simulink model "ARX_model_and_real_data"  (Simulink 5.0)
settings: Solver=ode45  StartTime=0.0  StopTime=10.0  RelTol=1e-3
settings Model: LastModifiedBy=Admin

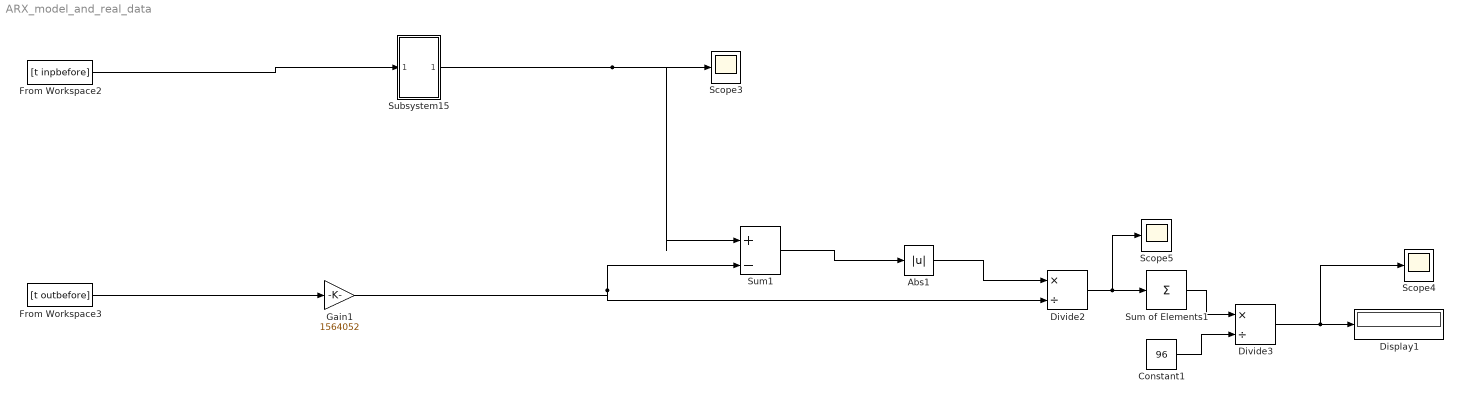
== system ARX_model_and_real_data ==
  Abs1 : Abs  SaturateOnIntegerOverflow=on
  Constant1 : Constant  Value=96
  Display1 : Display
  Divide2 : Product  Inputs=*/  ShowAdditionalParam=on  OutDataTypeMode=double  OutScaling=2^-10
  Divide3 : Product  Inputs=*/  ShowAdditionalParam=on  OutDataTypeMode=double  OutScaling=2^-10
  From Workspace2 : FromWorkspace  VariableName=[t inpbefore]  SampleTime=0
  From Workspace3 : FromWorkspace  VariableName=[t outbefore]  SampleTime=0
  Gain1 : Gain  Gain=1564052  SaturateOnIntegerOverflow=on
  Scope3 : Scope
  Scope4 : Scope
  Scope5 : Scope
      settings: SaveName=ScopeData2
  Subsystem15 : Subsystem
  Sum of Elements1 : Sum  Inputs=+  ShowAdditionalParam=on  OutDataTypeMode=double  OutScaling=2^-10
  Sum1 : Sum  Inputs=|+-  SaturateOnIntegerOverflow=on
  wires:
  From Workspace2/1 -> Subsystem15/1(In1)
  Subsystem15/1(Out1) -> Scope3/1, Sum1/1
  Sum1/1 -> Abs1/1
  Abs1/1 -> Divide2/1
  From Workspace3/1 -> Gain1/1
  Divide2/1 -> Sum of Elements1/1, Scope5/1
  Sum of Elements1/1 -> Divide3/1
  Divide3/1 -> Display1/1, Scope4/1
  Constant1/1 -> Divide3/2
  Gain1/1 -> Sum1/2, Divide2/2

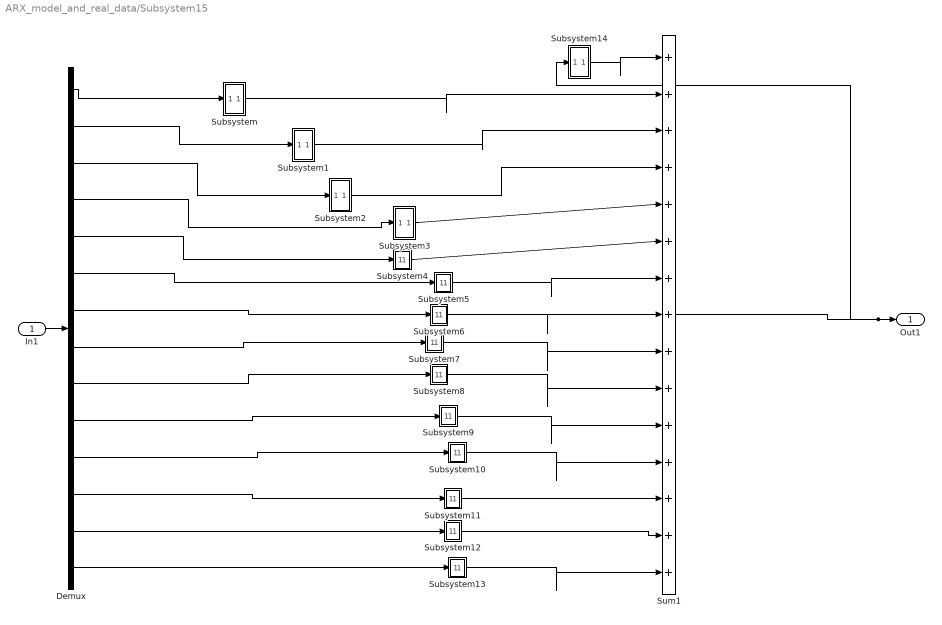
== system ARX_model_and_real_data/Subsystem15 ==
  In1 : Inport
  Demux : Demux  Outputs=14
  Subsystem : Subsystem
  Subsystem1 : Subsystem
  Subsystem10 : Subsystem
  Subsystem11 : Subsystem
  Subsystem12 : Subsystem
  Subsystem13 : Subsystem
  Subsystem14 : Subsystem
  Subsystem2 : Subsystem
  Subsystem3 : Subsystem
  Subsystem4 : Subsystem
  Subsystem5 : Subsystem
  Subsystem6 : Subsystem
  Subsystem7 : Subsystem
  Subsystem8 : Subsystem
  Subsystem9 : Subsystem
  Sum1 : Sum  Inputs=|+++++++++++++++  SaturateOnIntegerOverflow=on
  Out1 : Outport
  wires:
  Subsystem14/1(Out1) -> Sum1/1
  Sum1/1 -> Subsystem14/1(In1), Out1/1
  Demux/2 -> Subsystem1/1(In1)
  Demux/3 -> Subsystem2/1(In1)
  Demux/4 -> Subsystem3/1(In1)
  Demux/5 -> Subsystem4/1(In1)
  Demux/6 -> Subsystem5/1(In1)
  Demux/7 -> Subsystem6/1(In1)
  Demux/8 -> Subsystem7/1(In1)
  Demux/9 -> Subsystem8/1(In1)
  Demux/10 -> Subsystem9/1(In1)
  Demux/11 -> Subsystem10/1(In1)
  Demux/12 -> Subsystem11/1(In1)
  Demux/13 -> Subsystem12/1(In1)
  Demux/14 -> Subsystem13/1(In1)
  Subsystem13/1(Out1) -> Sum1/15
  Subsystem12/1(Out1) -> Sum1/14
  Subsystem11/1(Out1) -> Sum1/13
  Subsystem10/1(Out1) -> Sum1/12
  Subsystem9/1(Out1) -> Sum1/11
  Subsystem8/1(Out1) -> Sum1/10
  Subsystem7/1(Out1) -> Sum1/9
  Subsystem6/1(Out1) -> Sum1/8
  Subsystem5/1(Out1) -> Sum1/7
  Subsystem4/1(Out1) -> Sum1/6
  Subsystem3/1(Out1) -> Sum1/5
  Subsystem2/1(Out1) -> Sum1/4
  Subsystem1/1(Out1) -> Sum1/3
  Subsystem/1(Out1) -> Sum1/2
  Demux/1 -> Subsystem/1(In1)
  In1/1 -> Demux/1

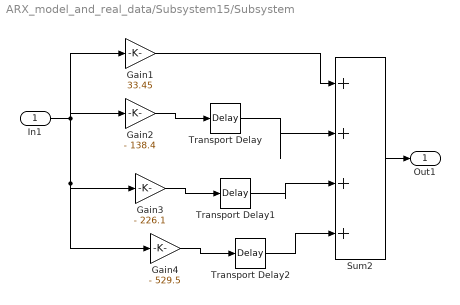
== system ARX_model_and_real_data/Subsystem15/Subsystem ==
  In1 : Inport
  Gain1 : Gain  Gain=33.45  SaturateOnIntegerOverflow=on
  Gain2 : Gain  Gain=- 138.4  SaturateOnIntegerOverflow=on
  Gain3 : Gain  Gain=- 226.1  SaturateOnIntegerOverflow=on
  Gain4 : Gain  Gain=- 529.5  SaturateOnIntegerOverflow=on
  Sum2 : Sum  Inputs=|++++  SaturateOnIntegerOverflow=on
  Transport Delay : TransportDelay
  Transport Delay1 : TransportDelay  DelayTime=2
  Transport Delay2 : TransportDelay  DelayTime=3
  Out1 : Outport
  wires:
  Gain4/1 -> Transport Delay2/1
  Transport Delay2/1 -> Sum2/4
  Gain2/1 -> Transport Delay/1
  Gain3/1 -> Transport Delay1/1
  Transport Delay/1 -> Sum2/2
  Transport Delay1/1 -> Sum2/3
  Gain1/1 -> Sum2/1
  In1/1 -> Gain2/1, Gain4/1, Gain3/1, Gain1/1
  Sum2/1 -> Out1/1

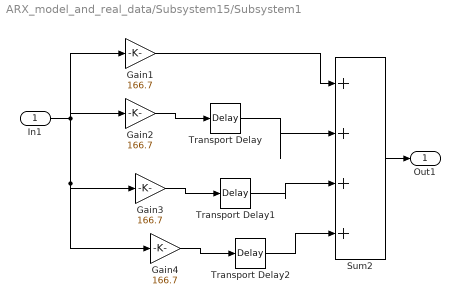
== system ARX_model_and_real_data/Subsystem15/Subsystem1 ==
  In1 : Inport
  Gain{1..4} (4 alike) : Gain  Gain=166.7  SaturateOnIntegerOverflow=on
  Sum2 : Sum  Inputs=|++++  SaturateOnIntegerOverflow=on
  Transport Delay : TransportDelay
  Transport Delay1 : TransportDelay  DelayTime=2
  Transport Delay2 : TransportDelay  DelayTime=3
  Out1 : Outport
  wires:
  Gain4/1 -> Transport Delay2/1
  Transport Delay2/1 -> Sum2/4
  Gain2/1 -> Transport Delay/1
  Gain3/1 -> Transport Delay1/1
  Transport Delay/1 -> Sum2/2
  Transport Delay1/1 -> Sum2/3
  Gain1/1 -> Sum2/1
  In1/1 -> Gain2/1, Gain4/1, Gain3/1, Gain1/1
  Sum2/1 -> Out1/1

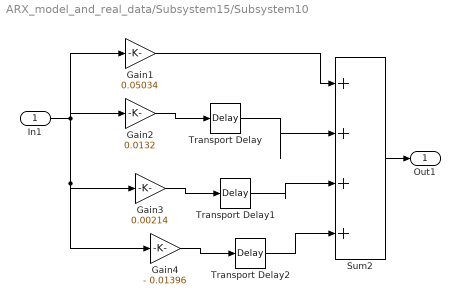
== system ARX_model_and_real_data/Subsystem15/Subsystem10 ==
  In1 : Inport
  Gain1 : Gain  Gain=0.05034  SaturateOnIntegerOverflow=on
  Gain2 : Gain  Gain=0.0132  SaturateOnIntegerOverflow=on
  Gain3 : Gain  Gain=0.00214  SaturateOnIntegerOverflow=on
  Gain4 : Gain  Gain=- 0.01396  SaturateOnIntegerOverflow=on
  Sum2 : Sum  Inputs=|++++  SaturateOnIntegerOverflow=on
  Transport Delay : TransportDelay
  Transport Delay1 : TransportDelay  DelayTime=2
  Transport Delay2 : TransportDelay  DelayTime=3
  Out1 : Outport
  wires:
  Gain4/1 -> Transport Delay2/1
  Transport Delay2/1 -> Sum2/4
  Gain2/1 -> Transport Delay/1
  Gain3/1 -> Transport Delay1/1
  Transport Delay/1 -> Sum2/2
  Transport Delay1/1 -> Sum2/3
  Gain1/1 -> Sum2/1
  In1/1 -> Gain2/1, Gain4/1, Gain3/1, Gain1/1
  Sum2/1 -> Out1/1

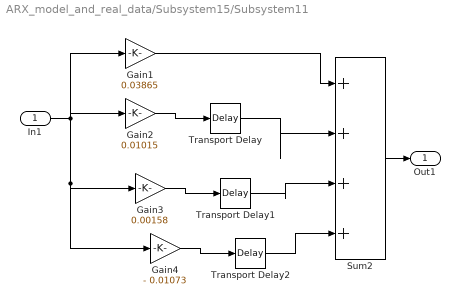
== system ARX_model_and_real_data/Subsystem15/Subsystem11 ==
  In1 : Inport
  Gain1 : Gain  Gain=0.03865  SaturateOnIntegerOverflow=on
  Gain2 : Gain  Gain=0.01015  SaturateOnIntegerOverflow=on
  Gain3 : Gain  Gain=0.00158  SaturateOnIntegerOverflow=on
  Gain4 : Gain  Gain=- 0.01073  SaturateOnIntegerOverflow=on
  Sum2 : Sum  Inputs=|++++  SaturateOnIntegerOverflow=on
  Transport Delay : TransportDelay
  Transport Delay1 : TransportDelay  DelayTime=2
  Transport Delay2 : TransportDelay  DelayTime=3
  Out1 : Outport
  wires:
  Gain4/1 -> Transport Delay2/1
  Transport Delay2/1 -> Sum2/4
  Gain2/1 -> Transport Delay/1
  Gain3/1 -> Transport Delay1/1
  Transport Delay/1 -> Sum2/2
  Transport Delay1/1 -> Sum2/3
  Gain1/1 -> Sum2/1
  In1/1 -> Gain2/1, Gain4/1, Gain3/1, Gain1/1
  Sum2/1 -> Out1/1

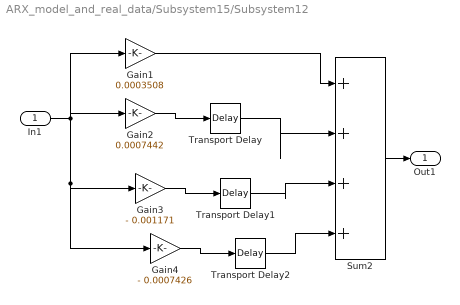
== system ARX_model_and_real_data/Subsystem15/Subsystem12 ==
  In1 : Inport
  Gain1 : Gain  Gain=0.0003508  SaturateOnIntegerOverflow=on
  Gain2 : Gain  Gain=0.0007442  SaturateOnIntegerOverflow=on
  Gain3 : Gain  Gain=- 0.001171  SaturateOnIntegerOverflow=on
  Gain4 : Gain  Gain=- 0.0007426  SaturateOnIntegerOverflow=on
  Sum2 : Sum  Inputs=|++++  SaturateOnIntegerOverflow=on
  Transport Delay : TransportDelay
  Transport Delay1 : TransportDelay  DelayTime=2
  Transport Delay2 : TransportDelay  DelayTime=3
  Out1 : Outport
  wires:
  Gain4/1 -> Transport Delay2/1
  Transport Delay2/1 -> Sum2/4
  Gain2/1 -> Transport Delay/1
  Gain3/1 -> Transport Delay1/1
  Transport Delay/1 -> Sum2/2
  Transport Delay1/1 -> Sum2/3
  Gain1/1 -> Sum2/1
  In1/1 -> Gain2/1, Gain4/1, Gain3/1, Gain1/1
  Sum2/1 -> Out1/1

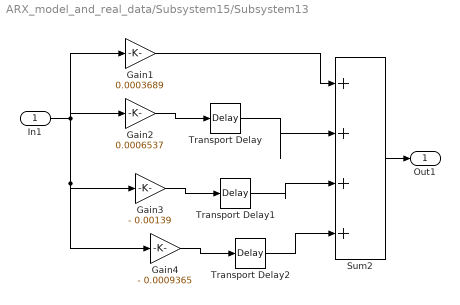
== system ARX_model_and_real_data/Subsystem15/Subsystem13 ==
  In1 : Inport
  Gain1 : Gain  Gain=0.0003689  SaturateOnIntegerOverflow=on
  Gain2 : Gain  Gain=0.0006537  SaturateOnIntegerOverflow=on
  Gain3 : Gain  Gain=- 0.00139  SaturateOnIntegerOverflow=on
  Gain4 : Gain  Gain=- 0.0009365  SaturateOnIntegerOverflow=on
  Sum2 : Sum  Inputs=|++++  SaturateOnIntegerOverflow=on
  Transport Delay : TransportDelay
  Transport Delay1 : TransportDelay  DelayTime=2
  Transport Delay2 : TransportDelay  DelayTime=3
  Out1 : Outport
  wires:
  Gain4/1 -> Transport Delay2/1
  Transport Delay2/1 -> Sum2/4
  Gain2/1 -> Transport Delay/1
  Gain3/1 -> Transport Delay1/1
  Transport Delay/1 -> Sum2/2
  Transport Delay1/1 -> Sum2/3
  Gain1/1 -> Sum2/1
  In1/1 -> Gain2/1, Gain4/1, Gain3/1, Gain1/1
  Sum2/1 -> Out1/1

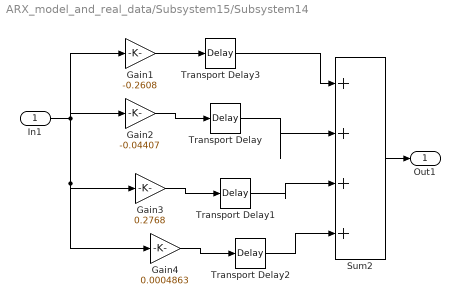
== system ARX_model_and_real_data/Subsystem15/Subsystem14 ==
  In1 : Inport
  Gain1 : Gain  Gain=-0.2608  SaturateOnIntegerOverflow=on
  Gain2 : Gain  Gain=-0.04407  SaturateOnIntegerOverflow=on
  Gain3 : Gain  Gain=0.2768  SaturateOnIntegerOverflow=on
  Gain4 : Gain  Gain=0.0004863  SaturateOnIntegerOverflow=on
  Sum2 : Sum  Inputs=|++++  SaturateOnIntegerOverflow=on
  Transport Delay : TransportDelay  DelayTime=2
  Transport Delay1 : TransportDelay  DelayTime=3
  Transport Delay2 : TransportDelay  DelayTime=4
  Transport Delay3 : TransportDelay
  Out1 : Outport
  wires:
  Gain4/1 -> Transport Delay2/1
  Transport Delay2/1 -> Sum2/4
  Gain2/1 -> Transport Delay/1
  Gain3/1 -> Transport Delay1/1
  Transport Delay/1 -> Sum2/2
  Transport Delay1/1 -> Sum2/3
  Gain1/1 -> Transport Delay3/1
  In1/1 -> Gain2/1, Gain4/1, Gain3/1, Gain1/1
  Sum2/1 -> Out1/1
  Transport Delay3/1 -> Sum2/1

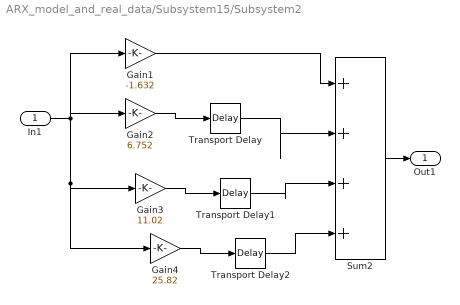
== system ARX_model_and_real_data/Subsystem15/Subsystem2 ==
  In1 : Inport
  Gain1 : Gain  Gain=-1.632  SaturateOnIntegerOverflow=on
  Gain2 : Gain  Gain=6.752  SaturateOnIntegerOverflow=on
  Gain3 : Gain  Gain=11.02  SaturateOnIntegerOverflow=on
  Gain4 : Gain  Gain=25.82  SaturateOnIntegerOverflow=on
  Sum2 : Sum  Inputs=|++++  SaturateOnIntegerOverflow=on
  Transport Delay : TransportDelay
  Transport Delay1 : TransportDelay  DelayTime=2
  Transport Delay2 : TransportDelay  DelayTime=3
  Out1 : Outport
  wires:
  Gain4/1 -> Transport Delay2/1
  Transport Delay2/1 -> Sum2/4
  Gain2/1 -> Transport Delay/1
  Gain3/1 -> Transport Delay1/1
  Transport Delay/1 -> Sum2/2
  Transport Delay1/1 -> Sum2/3
  Gain1/1 -> Sum2/1
  In1/1 -> Gain2/1, Gain4/1, Gain3/1, Gain1/1
  Sum2/1 -> Out1/1

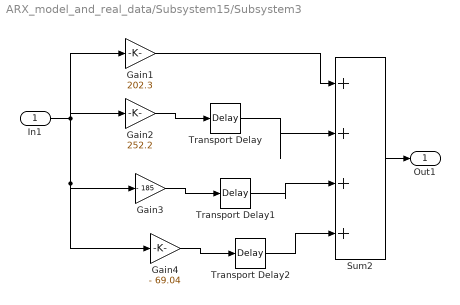
== system ARX_model_and_real_data/Subsystem15/Subsystem3 ==
  In1 : Inport
  Gain1 : Gain  Gain=202.3  SaturateOnIntegerOverflow=on
  Gain2 : Gain  Gain=252.2  SaturateOnIntegerOverflow=on
  Gain3 : Gain  Gain=- 185  SaturateOnIntegerOverflow=on
  Gain4 : Gain  Gain=- 69.04  SaturateOnIntegerOverflow=on
  Sum2 : Sum  Inputs=|++++  SaturateOnIntegerOverflow=on
  Transport Delay : TransportDelay
  Transport Delay1 : TransportDelay  DelayTime=2
  Transport Delay2 : TransportDelay  DelayTime=3
  Out1 : Outport
  wires:
  Gain4/1 -> Transport Delay2/1
  Transport Delay2/1 -> Sum2/4
  Gain2/1 -> Transport Delay/1
  Gain3/1 -> Transport Delay1/1
  Transport Delay/1 -> Sum2/2
  Transport Delay1/1 -> Sum2/3
  Gain1/1 -> Sum2/1
  In1/1 -> Gain2/1, Gain4/1, Gain3/1, Gain1/1
  Sum2/1 -> Out1/1

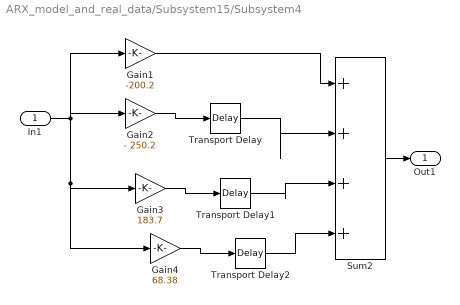
== system ARX_model_and_real_data/Subsystem15/Subsystem4 ==
  In1 : Inport
  Gain1 : Gain  Gain=-200.2  SaturateOnIntegerOverflow=on
  Gain2 : Gain  Gain=- 250.2  SaturateOnIntegerOverflow=on
  Gain3 : Gain  Gain=183.7  SaturateOnIntegerOverflow=on
  Gain4 : Gain  Gain=68.38  SaturateOnIntegerOverflow=on
  Sum2 : Sum  Inputs=|++++  SaturateOnIntegerOverflow=on
  Transport Delay : TransportDelay
  Transport Delay1 : TransportDelay  DelayTime=2
  Transport Delay2 : TransportDelay  DelayTime=3
  Out1 : Outport
  wires:
  Gain4/1 -> Transport Delay2/1
  Transport Delay2/1 -> Sum2/4
  Gain2/1 -> Transport Delay/1
  Gain3/1 -> Transport Delay1/1
  Transport Delay/1 -> Sum2/2
  Transport Delay1/1 -> Sum2/3
  Gain1/1 -> Sum2/1
  In1/1 -> Gain2/1, Gain4/1, Gain3/1, Gain1/1
  Sum2/1 -> Out1/1

== system ARX_model_and_real_data/Subsystem15/Subsystem5 ==
  In1 : Inport
  Gain1 : Gain  Gain=-1.473  SaturateOnIntegerOverflow=on
  Gain2 : Gain  Gain=- 1.841  SaturateOnIntegerOverflow=on
  Gain3 : Gain  Gain=1.351  SaturateOnIntegerOverflow=on
  Gain4 : Gain  Gain=0.5031  SaturateOnIntegerOverflow=on
  Sum2 : Sum  Inputs=|++++  SaturateOnIntegerOverflow=on
  Transport Delay : TransportDelay
  Transport Delay1 : TransportDelay  DelayTime=2
  Transport Delay2 : TransportDelay  DelayTime=3
  Out1 : Outport
  wires:
  Gain4/1 -> Transport Delay2/1
  Transport Delay2/1 -> Sum2/4
  Gain2/1 -> Transport Delay/1
  Gain3/1 -> Transport Delay1/1
  Transport Delay/1 -> Sum2/2
  Transport Delay1/1 -> Sum2/3
  Gain1/1 -> Sum2/1
  In1/1 -> Gain2/1, Gain4/1, Gain3/1, Gain1/1
  Sum2/1 -> Out1/1

== system ARX_model_and_real_data/Subsystem15/Subsystem6 ==
  In1 : Inport
  Gain1 : Gain  Gain=-5.55  SaturateOnIntegerOverflow=on
  Gain2 : Gain  Gain=24.53  SaturateOnIntegerOverflow=on
  Gain3 : Gain  Gain=39.93  SaturateOnIntegerOverflow=on
  Gain4 : Gain  Gain=93.38  SaturateOnIntegerOverflow=on
  Sum2 : Sum  Inputs=|++++  SaturateOnIntegerOverflow=on
  Transport Delay : TransportDelay
  Transport Delay1 : TransportDelay  DelayTime=2
  Transport Delay2 : TransportDelay  DelayTime=3
  Out1 : Outport
  wires:
  Gain4/1 -> Transport Delay2/1
  Transport Delay2/1 -> Sum2/4
  Gain2/1 -> Transport Delay/1
  Gain3/1 -> Transport Delay1/1
  Transport Delay/1 -> Sum2/2
  Transport Delay1/1 -> Sum2/3
  Gain1/1 -> Sum2/1
  In1/1 -> Gain2/1, Gain4/1, Gain3/1, Gain1/1
  Sum2/1 -> Out1/1

== system ARX_model_and_real_data/Subsystem15/Subsystem7 ==
  In1 : Inport
  Gain1 : Gain  Gain=0.0005023  SaturateOnIntegerOverflow=on
  Gain2 : Gain  Gain=- 0.0002562  SaturateOnIntegerOverflow=on
  Gain3 : Gain  Gain=0.0004082  SaturateOnIntegerOverflow=on
  Gain4 : Gain  Gain=- 0.0002853  SaturateOnIntegerOverflow=on
  Sum2 : Sum  Inputs=|++++  SaturateOnIntegerOverflow=on
  Transport Delay : TransportDelay
  Transport Delay1 : TransportDelay  DelayTime=2
  Transport Delay2 : TransportDelay  DelayTime=3
  Out1 : Outport
  wires:
  Gain4/1 -> Transport Delay2/1
  Transport Delay2/1 -> Sum2/4
  Gain2/1 -> Transport Delay/1
  Gain3/1 -> Transport Delay1/1
  Transport Delay/1 -> Sum2/2
  Transport Delay1/1 -> Sum2/3
  Gain1/1 -> Sum2/1
  In1/1 -> Gain2/1, Gain4/1, Gain3/1, Gain1/1
  Sum2/1 -> Out1/1

== system ARX_model_and_real_data/Subsystem15/Subsystem8 ==
  In1 : Inport
  Gain1 : Gain  Gain=0.0003028  SaturateOnIntegerOverflow=on
  Gain2 : Gain  Gain=0.0008254  SaturateOnIntegerOverflow=on
  Gain3 : Gain  Gain=- 0.0006172  SaturateOnIntegerOverflow=on
  Gain4 : Gain  Gain=0.0001375  SaturateOnIntegerOverflow=on
  Sum2 : Sum  Inputs=|++++  SaturateOnIntegerOverflow=on
  Transport Delay : TransportDelay
  Transport Delay1 : TransportDelay  DelayTime=2
  Transport Delay2 : TransportDelay  DelayTime=3
  Out1 : Outport
  wires:
  Gain4/1 -> Transport Delay2/1
  Transport Delay2/1 -> Sum2/4
  Gain2/1 -> Transport Delay/1
  Gain3/1 -> Transport Delay1/1
  Transport Delay/1 -> Sum2/2
  Transport Delay1/1 -> Sum2/3
  Gain1/1 -> Sum2/1
  In1/1 -> Gain2/1, Gain4/1, Gain3/1, Gain1/1
  Sum2/1 -> Out1/1

== system ARX_model_and_real_data/Subsystem15/Subsystem9 ==
  In1 : Inport
  Gain1 : Gain  Gain=-0.006094  SaturateOnIntegerOverflow=on
  Gain2 : Gain  Gain=- 0.001589  SaturateOnIntegerOverflow=on
  Gain3 : Gain  Gain=- 0.0002712  SaturateOnIntegerOverflow=on
  Gain4 : Gain  Gain=0.001686  SaturateOnIntegerOverflow=on
  Sum2 : Sum  Inputs=|++++  SaturateOnIntegerOverflow=on
  Transport Delay : TransportDelay
  Transport Delay1 : TransportDelay  DelayTime=2
  Transport Delay2 : TransportDelay  DelayTime=3
  Out1 : Outport
  wires:
  Gain4/1 -> Transport Delay2/1
  Transport Delay2/1 -> Sum2/4
  Gain2/1 -> Transport Delay/1
  Gain3/1 -> Transport Delay1/1
  Transport Delay/1 -> Sum2/2
  Transport Delay1/1 -> Sum2/3
  Gain1/1 -> Sum2/1
  In1/1 -> Gain2/1, Gain4/1, Gain3/1, Gain1/1
  Sum2/1 -> Out1/1
